simulink model "MPPT"  (R2021a)
settings: Solver=VariableStepAuto  StartTime=0.0  StopTime=10.0  RelTol=1e-3
libraries: simulink x1
settings Model: Creator=Harshitha  LastModifiedBy=Harshitha

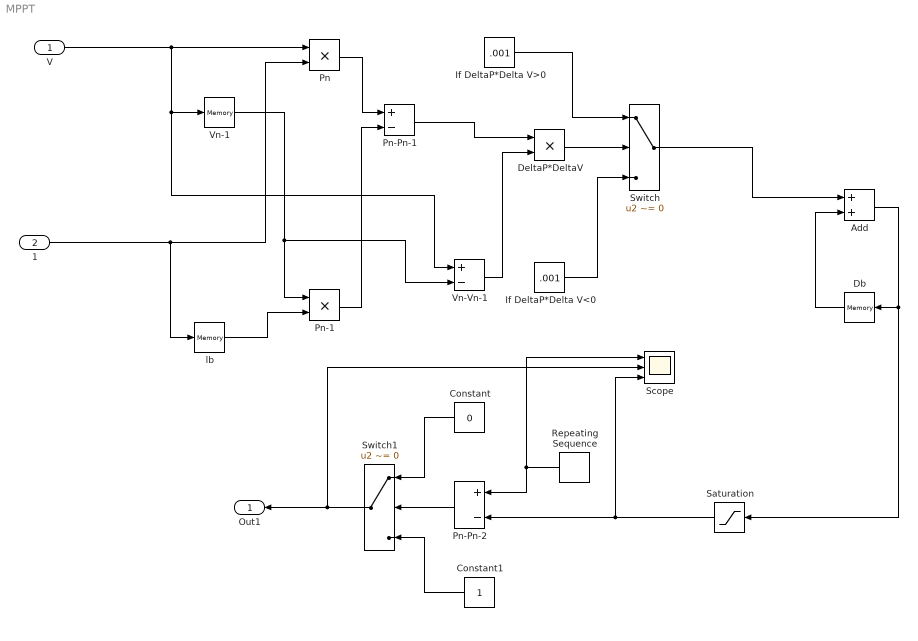
== system MPPT ==
  V : Inport
  1 : Inport  Port=2
  Add : Sum
  Constant : Constant  Value=0
  Constant1 : Constant
  Db : Memory  LinearizeAsDelay=on
  DeltaP*DeltaV : Product
  If DeltaP*Delta V<0 : Constant  Value=.001
  If DeltaP*Delta V>0 : Constant  Value=.001
  Pn : Product
  Pn-1 : Product
  Pn-Pn-1 : Sum  Inputs=+-
  Pn-Pn-2 : Sum  Inputs=+-
  Repeating Sequence : simulink/Sources/Repeating Sequence  rep_seq_t=[0 4e-4]  rep_seq_y=[0 1]
  Saturation : Saturate  UpperLimit=1
  Scope : Scope  NumInputPorts=3
  Switch : Switch  Criteria=u2 ~= 0  ZeroCross=off
  Switch1 : Switch  Criteria=u2 ~= 0
  Vn-1 : Memory
  Vn-Vn-1 : Sum  Inputs=+-
  lb : Memory
  Out1 : Outport
  wires:
  V/1 -> Pn/1, Vn-Vn-1/1, Vn-1/1
  1/1 -> Pn/2, lb/1
  Pn/1 -> Pn-Pn-1/1
  Pn-1/1 -> Pn-Pn-1/2
  Vn-1/1 -> Pn-1/1, Vn-Vn-1/2
  lb/1 -> Pn-1/2
  Pn-Pn-1/1 -> DeltaP*DeltaV/1
  Vn-Vn-1/1 -> DeltaP*DeltaV/2
  DeltaP*DeltaV/1 -> Switch/2
  If DeltaP*Delta V>0/1 -> Switch/1
  If DeltaP*Delta V<0/1 -> Switch/3
  Switch/1 -> Add/1
  Constant/1 -> Switch1/1
  Constant1/1 -> Switch1/3
  Pn-Pn-2/1 -> Switch1/2
  Repeating Sequence/1 -> Pn-Pn-2/1, Scope/1
  Saturation/1 -> Scope/3, Pn-Pn-2/2
  Add/1 -> Db/1, Saturation/1
  Db/1 -> Add/2
  Switch1/1 -> Scope/2, Out1/1
